simulink model "simulering"  (R2017a)
settings: Solver=VariableStepAuto  StartTime=0.0  StopTime=10.0  RelTol=1e-3
values from neighbouring files (symbols this model uses):
  Ad = 0.926549818887    [sysd.mat]    (also in trock.m = sysd.A)
  Bd = [-0.0657631580404 -0.00735568538738]    [sysd.mat]    (also in trock.m = [ sysd.B(5) sysd.B(6) ])
  Cd = [0.0055555252792 0.00510059552972]    [sysd.mat]    (also in trock.m = [ sysd.C(2); sysd.C(4) ])
  Dd = [-0.661477669827  -0.229336546845; -0.607310717919  -0.249936400478]    [sysd.mat]    (also in trock.m = [ sysd.D(2,5) sysd.D(2,6); sysd.D(4,5) sysd.D(4,6) ])
  E_new = Ed*pinv(Kd)    [MPC_model.m]    (also in sysd.mat = [0.000880261790191 0.00132062620896])
  Ts = 0.1    [sysd.mat]    (also in trock.m = 600)
undefined symbols (not defined in the file or in its folder): idss
libraries: slident x1
settings Model: Creator=nvink  LastModifiedBy=nvink

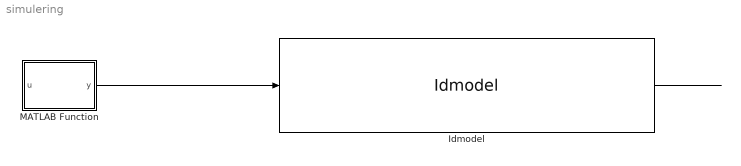
== system simulering ==
  Idmodel : slident/Models/Idmodel  sys=idss(Ad,Bd,Cd,Dd,E_new,Ts,1)  IC=0  noi=on  seed=[]
      settings: SourceProductName=System Identification Toolbox  SourceProductBaseCode=ID
  MATLAB Function : MATLAB Function  TreatAsAtomicUnit=on
  wires:
  MATLAB Function/1(y) -> Idmodel/1
  Idmodel/1 -> ?

== matlab function simulering/MATLAB Function ==
  data: u input; y output
function y = fcn(u)
workspace
%Solve a quadratic programming problem

%Variabels that we need to sort out.
% delta_p_0 d_hp U_bar_hp q_bar_p_hp
% 

% Variabels that we hare in the Matrix_op.m file
% Lambda_A Lambda_B Lambda_C Gamma Psi Phi Theta Omega Pi 
Matrix_op;
trock;                  %Load system matrices

delta_p_0 = 0.002;

d_hp = 0.05*90*ones(48,1);      % Small signal deviation of the Valves OD
U_bar_hp = 0.2*ones(48,1);      % Input pressure to ring pumps operating point
q_bar_p_hp = 1.4*ones(48,1);    % Flow operating point of the ring pumps


%%%%%%%%%%%%%%%%%% Generel QP %%%%%%%%%%%%%%%%%%
% 0.5*x'R*x+f'*x
%%%%%%%%%%%%%%%%%%%%%%%%%%%%%%%%%%%%%%%%%%%%%%%%%%%%%%%
%%%%%%%%%%%%%%%%%%%%% Constraint %%%%%%%%%%%%%%%%%%%%%%
%%%%%%%%%%%%%%%%%%%%%%%%%%%%%%%%%%%%%%%%%%%%%%%%%%%%%%%

% Output constraint
y_low = -0.0755*ones(48,1);         % Lower bound small deviation for Pressure PMA
y_high = 0.0245*ones(48,1);         % Upper bound small deviation for Pressure PMA

% Pressure operating point of the PMA end-users
y_bar = [0.1562; 0.0991 ;0.1562; 0.0991 ;0.1562; 0.0991 ;0.1562; 0.0991 ;0.1562; 0.0991 ;0.1562; 0.0991 ;
        0.1562; 0.0991 ;0.1562; 0.0991 ;0.1562; 0.0991 ;0.1562; 0.0991 ;0.1562; 0.0991 ;0.1562; 0.0991 ;
        0.1562; 0.0991 ;0.1562; 0.0991 ;0.1562; 0.0991 ;0.1562; 0.0991 ;0.1562; 0.0991 ;0.1562; 0.0991 ;
        0.1562; 0.0991 ;0.1562; 0.0991 ;0.1562; 0.0991 ;0.1562; 0.0991 ;0.1562; 0.0991 ;0.1562; 0.0991];    


y1 = y_low - y_bar - Theta*Phi*delta_p_0-(Theta*Psi+Pi)*d_hp;
y2 = y_high - y_bar - Theta*Phi*delta_p_0-(Theta*Psi+Pi)*d_hp;
L_y = Theta*Gamma+Omega;

% State constraint
x_low = -0.077*ones(24,1);
x_high = 0.033*ones(24,1);
x_bar = 0.127*ones(24,1);

dalta_p_wt_1 = x_low-x_bar - Phi*delta_p_0 - Psi*d_hp;
dalta_p_wt_2 = x_high-x_bar - Phi*delta_p_0 - Psi*d_hp;

% input constraint 
u_low = 0;
u_high = 1;

%%%%%%%%%%%%%%%%%%%%%%%%%%%%%%%%%%%%%%%%%%%%%%%%%%%%%%%
%%%%%%%%%%%%%%%%%% Setting up the QP %%%%%%%%%%%%%%%%%% 
%%%%%%%%%%%%%%%%%%%%%%%%%%%%%%%%%%%%%%%%%%%%%%%%%%%%%%%

R = 2*(Lambda_A + Lambda_C*Gamma); 

f = U_bar_hp'*(Lambda_A+Lambda_C*Gamma)+d_hp'*(Lambda_B+Lambda_C*Psi)'+delta_p_0*(Lambda_C*Phi)'+q_bar_p_hp';

A = [-L_y; L_y; -Gamma; Gamma];
b = [y1; y2; dalta_p_wt_1; dalta_p_wt_2];

lb = u_low*ones(48,1);
ub = u_high*ones(48,1);

%options = optimoptions('Display','iter-detailed');%quadprog

options = optimoptions('quadprog','Display','iter-detailed')
[u_hp,cost,output,lambda] = ...
   quadprog(R,f,[],[],[],[],lb,ub,[],options);

u_hp,cost

y = u;
